simulink model "IMU"  (R2021a)
settings: Solver=VariableStepAuto  StartTime=0.0  StopTime=10.0  RelTol=1e-3
values from neighbouring files (symbols this model uses):
  Sensor_err = read_sensor_data    [main.m]
libraries: dspsrcs4 x13, sharedtransform x1, simulink_extras x1
settings Model: Creator=mojta  LastModifiedBy=mojta

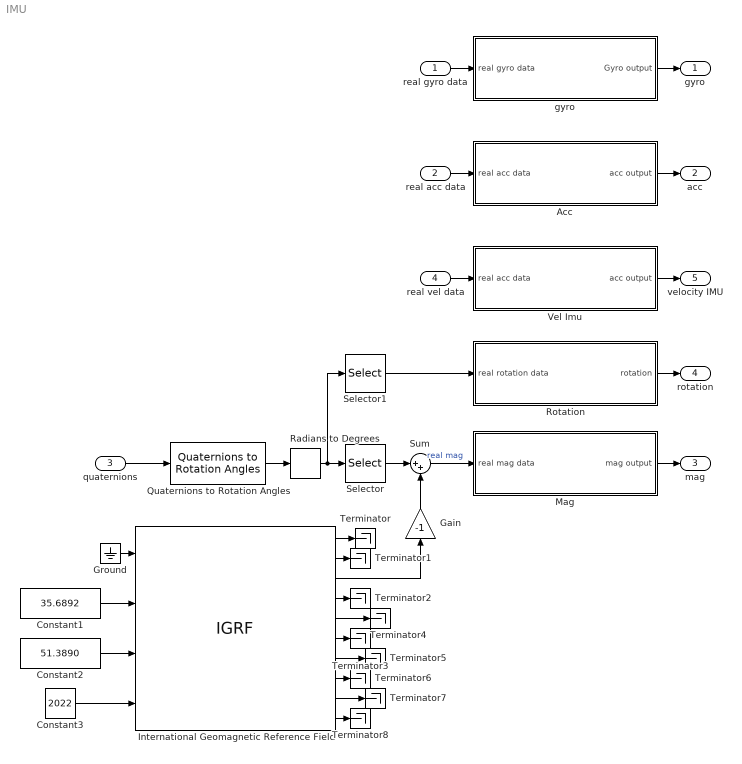
== system IMU ==
  real gyro data : Inport  PortDimensions=3
  real acc data : Inport  Port=2  PortDimensions=3
  quaternions : Inport  Port=3  PortDimensions=4
  real vel data : Inport  Port=4  PortDimensions=3
  Acc : Subsystem
  Constant1 : Constant  Value=35.6892
  Constant2 : Constant  Value=51.3890
  Constant3 : Constant  Value=2022
  Gain : Gain  Gain=-1
  Ground : Ground
  International Geomagnetic Reference Field : IGRF  month=January  day=1  year=2020
      settings: AttributesFormatString=%<generation>
  Mag : Subsystem
  Quaternions to Rotation Angles : sharedtransform/Quaternions to Rotation Angles  rotationOrder=ZYX  aMode=aMode
      settings: SourceProductBaseCode=AE,PW,DR,MT,UV,VE
  Radians to Degrees : simulink_extras/Transformations/Radians to Degrees
  Rotation : Subsystem
  Selector : Selector  InputPortWidth=3  IndexOptions=Index vector (dialog)  Indices=1  OutputSizes=1
  Selector1 : Selector  InputPortWidth=3  IndexOptions=Index vector (dialog)  Indices=[3 2 1]  OutputSizes=1
  Sum : Sum  Inputs=|++
  Terminator{,1..8} (9 alike) : Terminator
  Vel Imu : Subsystem
  gyro : Subsystem
  "gyro " : Outport
  acc : Outport  Port=2
  mag : Outport  Port=3
  rotation : Outport  Port=4
  velocity IMU : Outport  Port=5
  wires:
  real gyro data/1 -> gyro/1(real gyro data)
  gyro/1(Gyro output) -> "gyro "/1
  real acc data/1 -> Acc/1(real acc data)
  Acc/1(acc output) -> acc/1
  quaternions/1 -> Quaternions to Rotation Angles/1
  Mag/1(mag output) -> mag/1
  Quaternions to Rotation Angles/1 -> Radians to Degrees/1
  Constant2/1 -> International Geomagnetic Reference Field/3
  Constant3/1 -> International Geomagnetic Reference Field/4
  Constant1/1 -> International Geomagnetic Reference Field/2
  Ground/1 -> International Geomagnetic Reference Field/1
  International Geomagnetic Reference Field/3 -> Gain/1
  Gain/1 -> Sum/2
  Sum/1 -> Mag/1(real mag data)  "real mag"
  International Geomagnetic Reference Field/1 -> Terminator/1
  International Geomagnetic Reference Field/2 -> Terminator1/1
  International Geomagnetic Reference Field/4 -> Terminator2/1
  International Geomagnetic Reference Field/6 -> Terminator3/1
  International Geomagnetic Reference Field/5 -> Terminator4/1
  International Geomagnetic Reference Field/7 -> Terminator5/1
  International Geomagnetic Reference Field/8 -> Terminator6/1
  International Geomagnetic Reference Field/9 -> Terminator7/1
  International Geomagnetic Reference Field/10 -> Terminator8/1
  Selector/1 -> Sum/1
  Radians to Degrees/1 -> Selector1/1, Selector/1
  Selector1/1 -> Rotation/1(real rotation data)
  Rotation/1(rotation) -> rotation/1
  Vel Imu/1(acc output) -> velocity IMU/1
  real vel data/1 -> Vel Imu/1(real acc data)

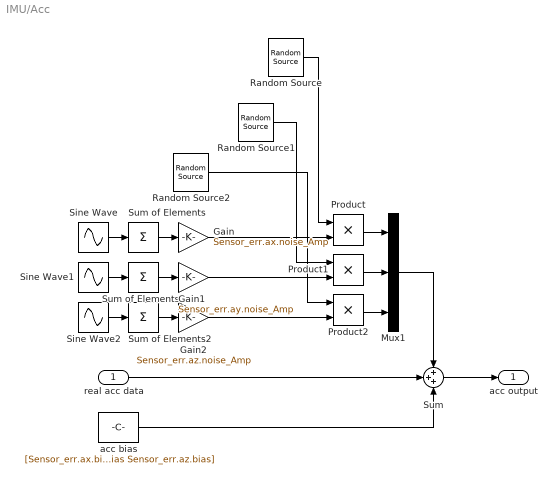
== system IMU/Acc ==
  real acc data : Inport
  Gain : Gain  Gain=Sensor_err.ax.noise_Amp
  Gain1 : Gain  Gain=Sensor_err.ay.noise_Amp
  Gain2 : Gain  Gain=Sensor_err.az.noise_Amp
  Mux1 : Mux  Inputs=3
  Product : Product
  Product1 : Product
  Product2 : Product
  Random Source : dspsrcs4/Random Source  SrcType=Uniform  NormMethod=Ziggurat  CltLength=12  MinVal=0  MaxVal=1  MeanVal=0  VarVal=1  RepMode=Not repeatable  rawSeed=1  IsInherit=off  SampMode=Discrete  SampTime=1  SampFrame=1  DataType=Double  OutComplex=Real  OutputFrames=off
  Random Source1 : dspsrcs4/Random Source  SrcType=Uniform  NormMethod=Ziggurat  CltLength=12  MinVal=0  MaxVal=1  MeanVal=0  VarVal=1  RepMode=Not repeatable  rawSeed=1  IsInherit=off  SampMode=Discrete  SampTime=1  SampFrame=1  DataType=Double  OutComplex=Real  OutputFrames=off
  Random Source2 : dspsrcs4/Random Source  SrcType=Uniform  NormMethod=Ziggurat  CltLength=12  MinVal=0  MaxVal=1  MeanVal=0  VarVal=1  RepMode=Not repeatable  rawSeed=1  IsInherit=off  SampMode=Discrete  SampTime=1  SampFrame=1  DataType=Double  OutComplex=Real  OutputFrames=off
  Sine Wave : Sin  Frequency=2*pi*Sensor_err.ax.freqs  SampleTime=0
  Sine Wave1 : Sin  Frequency=2*pi*Sensor_err.ay.freqs  SampleTime=0
  Sine Wave2 : Sin  Frequency=2*pi*Sensor_err.az.freqs  SampleTime=0
  Sum : Sum  Inputs=3
  Sum of Elements : Sum  Inputs=+
  Sum of Elements1 : Sum  Inputs=+
  Sum of Elements2 : Sum  Inputs=+
  acc bias : Constant  Value=[Sensor_err.ax.bias Sensor_err.ay.bias Sensor_err.az.bias]
  acc output : Outport
  wires:
  Sine Wave1/1 -> Sum of Elements1/1
  Sine Wave2/1 -> Sum of Elements2/1
  Sum/1 -> acc output/1
  real acc data/1 -> Sum/2
  Sine Wave/1 -> Sum of Elements/1
  Sum of Elements/1 -> Gain/1
  Sum of Elements1/1 -> Gain1/1
  Gain2/1 -> Product2/2
  acc bias/1 -> Sum/3
  Sum of Elements2/1 -> Gain2/1
  Gain1/1 -> Product1/2
  Gain/1 -> Product/2
  Product1/1 -> Mux1/2
  Mux1/1 -> Sum/1
  Random Source2/1 -> Product2/1
  Product2/1 -> Mux1/3
  Random Source1/1 -> Product1/1
  Product/1 -> Mux1/1
  Random Source/1 -> Product/1

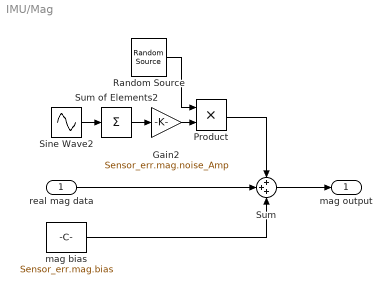
== system IMU/Mag ==
  real mag data : Inport
  Gain2 : Gain  Gain=Sensor_err.mag.noise_Amp
  Product : Product
  Random Source : dspsrcs4/Random Source  SrcType=Uniform  NormMethod=Ziggurat  CltLength=12  MinVal=0  MaxVal=1  MeanVal=0  VarVal=1  RepMode=Not repeatable  rawSeed=1  IsInherit=off  SampMode=Discrete  SampTime=1  SampFrame=1  DataType=Double  OutComplex=Real  OutputFrames=off
  Sine Wave2 : Sin  Frequency=2*pi*Sensor_err.mag.freqs  SampleTime=0
  Sum : Sum  Inputs=3
  Sum of Elements2 : Sum  Inputs=+
  mag bias : Constant  Value=Sensor_err.mag.bias
  mag output : Outport
  wires:
  Sum of Elements2/1 -> Gain2/1
  mag bias/1 -> Sum/3
  real mag data/1 -> Sum/2
  Sum/1 -> mag output/1
  Sine Wave2/1 -> Sum of Elements2/1
  Gain2/1 -> Product/2
  Random Source/1 -> Product/1
  Product/1 -> Sum/1

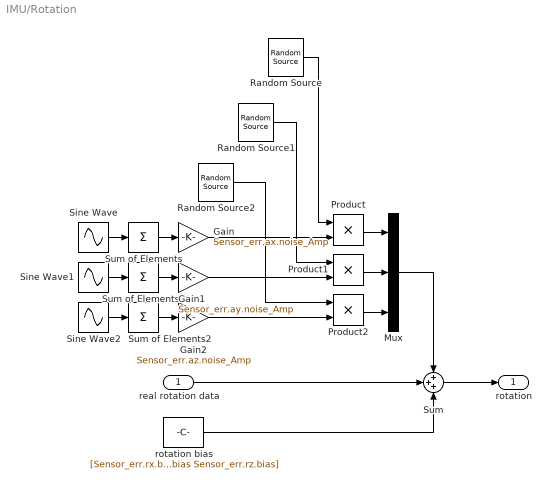
== system IMU/Rotation ==
  real rotation data : Inport
  Gain : Gain  Gain=Sensor_err.ax.noise_Amp
  Gain1 : Gain  Gain=Sensor_err.ay.noise_Amp
  Gain2 : Gain  Gain=Sensor_err.az.noise_Amp
  Mux : Mux  Inputs=3
  Product : Product
  Product1 : Product
  Product2 : Product
  Random Source : dspsrcs4/Random Source  SrcType=Uniform  NormMethod=Ziggurat  CltLength=12  MinVal=0  MaxVal=1  MeanVal=0  VarVal=1  RepMode=Not repeatable  rawSeed=1  IsInherit=off  SampMode=Discrete  SampTime=1  SampFrame=1  DataType=Double  OutComplex=Real  OutputFrames=off
  Random Source1 : dspsrcs4/Random Source  SrcType=Uniform  NormMethod=Ziggurat  CltLength=12  MinVal=0  MaxVal=1  MeanVal=0  VarVal=1  RepMode=Not repeatable  rawSeed=1  IsInherit=off  SampMode=Discrete  SampTime=1  SampFrame=1  DataType=Double  OutComplex=Real  OutputFrames=off
  Random Source2 : dspsrcs4/Random Source  SrcType=Uniform  NormMethod=Ziggurat  CltLength=12  MinVal=0  MaxVal=1  MeanVal=0  VarVal=1  RepMode=Not repeatable  rawSeed=1  IsInherit=off  SampMode=Discrete  SampTime=1  SampFrame=1  DataType=Double  OutComplex=Real  OutputFrames=off
  Sine Wave : Sin  Frequency=2*pi*Sensor_err.rx.freqs  SampleTime=0
  Sine Wave1 : Sin  Frequency=2*pi*Sensor_err.ry.freqs  SampleTime=0
  Sine Wave2 : Sin  Frequency=2*pi*Sensor_err.rz.freqs  SampleTime=0
  Sum : Sum  Inputs=3
  Sum of Elements : Sum  Inputs=+
  Sum of Elements1 : Sum  Inputs=+
  Sum of Elements2 : Sum  Inputs=+
  rotation bias : Constant  Value=[Sensor_err.rx.bias Sensor_err.ry.bias Sensor_err.rz.bias]
  rotation : Outport
  wires:
  Gain/1 -> Product/2
  Gain1/1 -> Product1/2
  Sum of Elements2/1 -> Gain2/1
  rotation bias/1 -> Sum/3
  Gain2/1 -> Product2/2
  Sum of Elements1/1 -> Gain1/1
  Sum of Elements/1 -> Gain/1
  Sine Wave/1 -> Sum of Elements/1
  real rotation data/1 -> Sum/2
  Sum/1 -> rotation/1
  Sine Wave2/1 -> Sum of Elements2/1
  Sine Wave1/1 -> Sum of Elements1/1
  Mux/1 -> Sum/1
  Random Source/1 -> Product/1
  Product1/1 -> Mux/2
  Product/1 -> Mux/1
  Product2/1 -> Mux/3
  Random Source1/1 -> Product1/1
  Random Source2/1 -> Product2/1

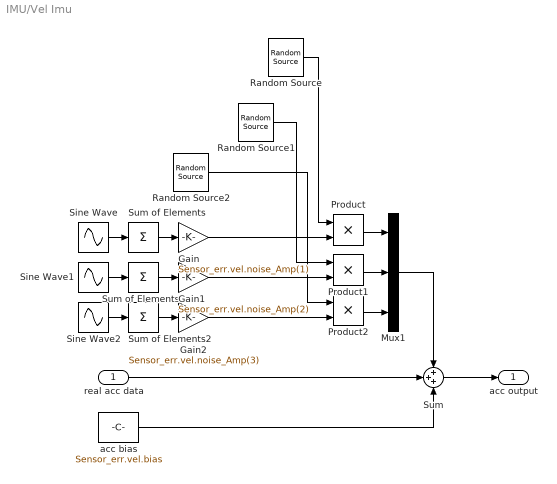
== system IMU/Vel Imu ==
  real acc data : Inport
  Gain : Gain  Gain=Sensor_err.vel.noise_Amp(1)
  Gain1 : Gain  Gain=Sensor_err.vel.noise_Amp(2)
  Gain2 : Gain  Gain=Sensor_err.vel.noise_Amp(3)
  Mux1 : Mux  Inputs=3
  Product : Product
  Product1 : Product
  Product2 : Product
  Random Source : dspsrcs4/Random Source  SrcType=Uniform  NormMethod=Ziggurat  CltLength=12  MinVal=0  MaxVal=1  MeanVal=0  VarVal=1  RepMode=Not repeatable  rawSeed=1  IsInherit=off  SampMode=Discrete  SampTime=1  SampFrame=1  DataType=Double  OutComplex=Real  OutputFrames=off
  Random Source1 : dspsrcs4/Random Source  SrcType=Uniform  NormMethod=Ziggurat  CltLength=12  MinVal=0  MaxVal=1  MeanVal=0  VarVal=1  RepMode=Not repeatable  rawSeed=1  IsInherit=off  SampMode=Discrete  SampTime=1  SampFrame=1  DataType=Double  OutComplex=Real  OutputFrames=off
  Random Source2 : dspsrcs4/Random Source  SrcType=Uniform  NormMethod=Ziggurat  CltLength=12  MinVal=0  MaxVal=1  MeanVal=0  VarVal=1  RepMode=Not repeatable  rawSeed=1  IsInherit=off  SampMode=Discrete  SampTime=1  SampFrame=1  DataType=Double  OutComplex=Real  OutputFrames=off
  Sine Wave : Sin  Frequency=2*pi*Sensor_err.vel.freqs_x  SampleTime=0
  Sine Wave1 : Sin  Frequency=2*pi*Sensor_err.vel.freqs_y  SampleTime=0
  Sine Wave2 : Sin  Frequency=2*pi*Sensor_err.vel.freqs_z  SampleTime=0
  Sum : Sum  Inputs=3
  Sum of Elements : Sum  Inputs=+
  Sum of Elements1 : Sum  Inputs=+
  Sum of Elements2 : Sum  Inputs=+
  acc bias : Constant  Value=Sensor_err.vel.bias
  acc output : Outport
  wires:
  Random Source/1 -> Product/1
  Product/1 -> Mux1/1
  Random Source1/1 -> Product1/1
  Product2/1 -> Mux1/3
  Random Source2/1 -> Product2/1
  Mux1/1 -> Sum/1
  Product1/1 -> Mux1/2
  Gain/1 -> Product/2
  Gain1/1 -> Product1/2
  Sum of Elements2/1 -> Gain2/1
  acc bias/1 -> Sum/3
  Gain2/1 -> Product2/2
  Sum of Elements1/1 -> Gain1/1
  Sum of Elements/1 -> Gain/1
  Sine Wave/1 -> Sum of Elements/1
  real acc data/1 -> Sum/2
  Sum/1 -> acc output/1
  Sine Wave2/1 -> Sum of Elements2/1
  Sine Wave1/1 -> Sum of Elements1/1

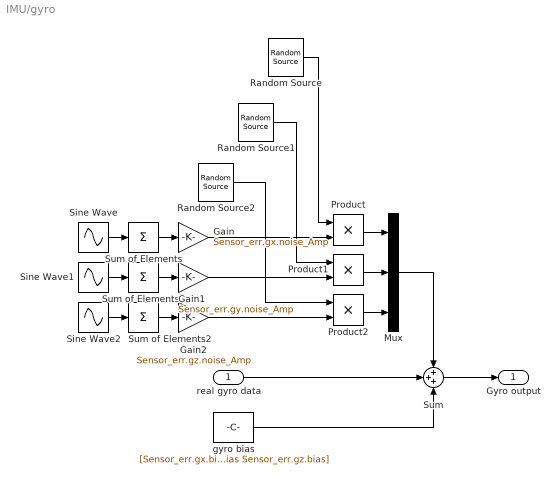
== system IMU/gyro ==
  real gyro data : Inport
  Gain : Gain  Gain=Sensor_err.gx.noise_Amp
  Gain1 : Gain  Gain=Sensor_err.gy.noise_Amp
  Gain2 : Gain  Gain=Sensor_err.gz.noise_Amp
  Mux : Mux  Inputs=3
  Product : Product
  Product1 : Product
  Product2 : Product
  Random Source : dspsrcs4/Random Source  SrcType=Uniform  NormMethod=Ziggurat  CltLength=12  MinVal=0  MaxVal=1  MeanVal=0  VarVal=1  RepMode=Not repeatable  rawSeed=1  IsInherit=off  SampMode=Discrete  SampTime=1  SampFrame=1  DataType=Double  OutComplex=Real  OutputFrames=off
  Random Source1 : dspsrcs4/Random Source  SrcType=Uniform  NormMethod=Ziggurat  CltLength=12  MinVal=0  MaxVal=1  MeanVal=0  VarVal=1  RepMode=Not repeatable  rawSeed=1  IsInherit=off  SampMode=Discrete  SampTime=1  SampFrame=1  DataType=Double  OutComplex=Real  OutputFrames=off
  Random Source2 : dspsrcs4/Random Source  SrcType=Uniform  NormMethod=Ziggurat  CltLength=12  MinVal=0  MaxVal=1  MeanVal=0  VarVal=1  RepMode=Not repeatable  rawSeed=1  IsInherit=off  SampMode=Discrete  SampTime=1  SampFrame=1  DataType=Double  OutComplex=Real  OutputFrames=off
  Sine Wave : Sin  Frequency=2*pi*Sensor_err.gx.freqs  SampleTime=0
  Sine Wave1 : Sin  Frequency=2*pi*Sensor_err.gy.freqs  SampleTime=0
  Sine Wave2 : Sin  Frequency=2*pi*Sensor_err.gz.freqs  SampleTime=0
  Sum : Sum  Inputs=3
  Sum of Elements : Sum  Inputs=+
  Sum of Elements1 : Sum  Inputs=+
  Sum of Elements2 : Sum  Inputs=+
  gyro bias : Constant  Value=[Sensor_err.gx.bias Sensor_err.gy.bias Sensor_err.gz.bias]
  Gyro output : Outport
  wires:
  Sum of Elements2/1 -> Gain2/1
  gyro bias/1 -> Sum/3
  Sum of Elements1/1 -> Gain1/1
  Sum of Elements/1 -> Gain/1
  Sine Wave/1 -> Sum of Elements/1
  real gyro data/1 -> Sum/2
  Sum/1 -> Gyro output/1
  Sine Wave2/1 -> Sum of Elements2/1
  Sine Wave1/1 -> Sum of Elements1/1
  Gain/1 -> Product/2
  Product1/1 -> Mux/2
  Mux/1 -> Sum/1
  Gain2/1 -> Product2/2
  Random Source2/1 -> Product2/1
  Product2/1 -> Mux/3
  Random Source1/1 -> Product1/1
  Gain1/1 -> Product1/2
  Product/1 -> Mux/1
  Random Source/1 -> Product/1
